simulink model "smc_AMB_digital_v2"  (R2025b)
settings: Solver=FixedStepAuto  StartTime=0.0  StopTime=2.9  FixedStep=0.0001  RelTol=1e-3
values from neighbouring files (symbols this model uses):
  a = -0.315/2    (= -0.1575)    [configura_planta_simulacao2.m]
  alpha = 0.8819    [configura_planta_simulacao2.m]
  Ar = 2*0.0077*0.0165*cos(pi/8)    [configura_planta_simulacao2.m]
  b = 0.315/2    (= 0.1575)    [configura_planta_simulacao2.m]
  Ix = 1/12*m*(L^2 +3*(dia/2)^2)    (= 0.0133460782333)    [configura_planta_simulacao2.m]
  Iy = Ix    (= 0.0133460782333)    [configura_planta_simulacao2.m]
  Iz = m*(dia/2)^2/2    (= 2.54898e-05)    [configura_planta_simulacao2.m]
  Kd_pid = 49    [configura_planta_simulacao2.m]
  Ki_pid = 4e4    (= 40000)    [configura_planta_simulacao2.m]
  Kp_pid = 1.2e4    (= 12000)    [configura_planta_simulacao2.m]
  m = 1    [configura_planta_simulacao2.m]
  mi0 = pi*4e-7    (= 1.25663706144e-06)    [configura_planta_simulacao2.m]
  n = 260    [configura_planta_simulacao2.m]    (also in plot_simu.m = round(numel(xs) * alvo/ppv))
  omega = 0    [configura_planta_simulacao2.m]
  Ts = 1e-4    (= 0.0001)    [configura_planta_simulacao2.m]    (also in smc_mancal_simulacao.m = single(1e-4))
  U = [IneS(2,3)+b*CM(2)*mT, IneS(3,1)-b*CM(1)*mT ... (first row only)    [configura_planta_simulacao2.m]
  y0 = -5e-4    (= -0.0005)    [configura_planta_simulacao2.m]
undefined symbols (not defined in the file or in its folder): magnitude
libraries: simulink x4
settings Model: NumberOfSteps=5  Creator=thaty  LastModifiedBy=thaty
settings RTWCC: GPUComputeCapability=3.5

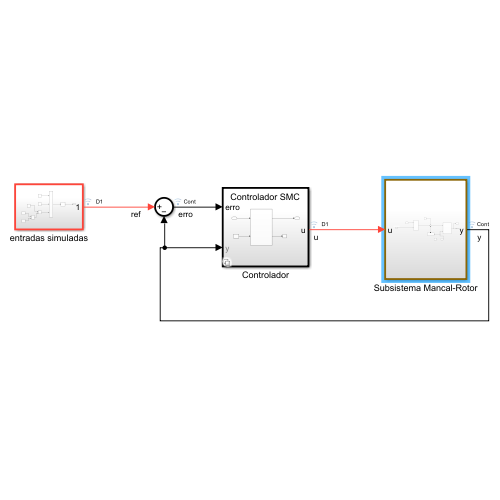
[thumbnail: Simulink's stored preview of the top-level diagram]
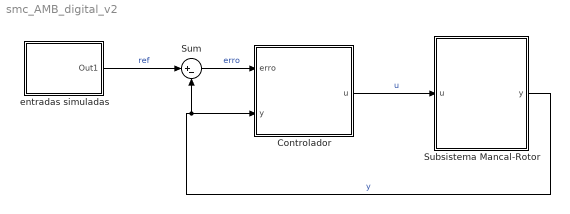
== system smc_AMB_digital_v2 ==
  Controlador : Subsystem  Variant=on
  Subsistema Mancal-Rotor : Subsystem
  Sum : Sum  Inputs=|+-
  entradas simuladas : Subsystem
  wires:
  Sum/1 -> Controlador/1(erro)  "erro"
  entradas simuladas/1(Out1) -> Sum/1  "ref"
  Subsistema Mancal-Rotor/1(y) -> Controlador/2(y), Sum/2  "y"
  Controlador/1(u) -> Subsistema Mancal-Rotor/1(u)  "u"

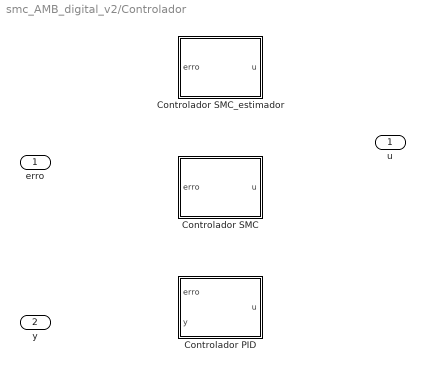
== system smc_AMB_digital_v2/Controlador ==
  erro : Inport
  y : Inport  Port=2
  Controlador PID : Subsystem  VariantControl=Type==1
  Controlador SMC : Subsystem  VariantControl=Type==2
  Controlador SMC_estimador : Subsystem  VariantControl=Type==3
  u : Outport

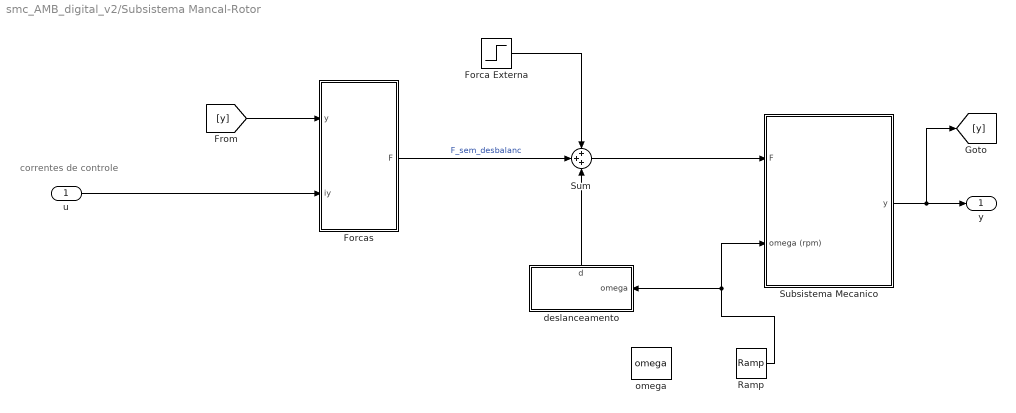
== system smc_AMB_digital_v2/Subsistema Mancal-Rotor ==
  note: correntes de controle
  u : Inport
  Forca Externa : Step  Time=2  After=0  SampleTime=0
  Forcas : Subsystem
  Ramp : simulink/Sources/Ramp  slope=10000  start=0  InitialOutput=0
  Subsistema Mecanico : Subsystem
  Sum : Sum  Inputs=+++
  deslanceamento : Subsystem
      settings: PortSchema="{\"entries\":[{\"content\":{\"sides\":[{\"content\":{},\"type\":\"ConnectorPlacement.EquallySpacedRectSide\",\"uuid\":\"45b55e67-a5ed-4805-aab1-a3da632aa8db\"},{\"content\":{\"connectorIds\":[\"In1\"],\"side\":\"RIGHT\"},\"type\":\"ConnectorPlacement.EquallySpacedRectSide\",\"uuid\":\"03c95f23-bcb1-4d33-8836-c97663662569\"},{\"content\":{\"connectorIds\":[\"Out1\"],\"side\":\"TOP\"},\"type\":\"ConnectorPlacement.EquallySpacedRectSide\",\"uuid\":\"b340f43e-95d2-40b9-ae6d-e83cbb66ff43\"}]},\"type\":\"ConnectorPlacement.EquallySpacedConnector\",\"uuid\":\"389c9e54-a030-42d8-804b-2d0e7948bbc4\"}],\"packageUris\":[\"http://schema.mathworks.com/mf0/Connector/R2020b\"],\"version\":\"1.0\"}"
  omega : Constant  Value=omega
  y : Outport
  wires:
  [y] -> Forcas/1(y)
  Forcas/1(F) -> Sum/2  "F_sem_desbalanc"
  Sum/1 -> Subsistema Mecanico/1(F)
  deslanceamento/1(d) -> Sum/3
  Subsistema Mecanico/1(y) -> [y], y/1
  Forca Externa/1 -> Sum/1
  Ramp/1 -> deslanceamento/1(omega), Subsistema Mecanico/2(omega (rpm))
  u/1 -> Forcas/2(iy)

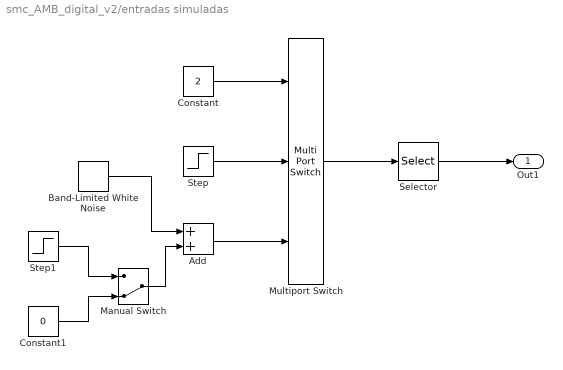
== system smc_AMB_digital_v2/entradas simuladas ==
  Add : Sum
  Band-Limited White Noise : simulink/Sources/Band-Limited White Noise  Cov=1e-14  Ts=0.0001  seed=[23341]
  Constant : Constant  Value=2
  Constant1 : Constant  Value=0
  Manual Switch : ManualSwitch  CurrentSetting=0
  Multiport Switch : MultiPortSwitch  Inputs=2  SaturateOnIntegerOverflow=off  InputSameDT=off
  Selector : Selector  InputPortWidth=1  IndexOptions=Index vector (dialog)  Indices=[1 1 1 1]  OutputSizes=1
  Step : Step  Before=y0  After=0  SampleTime=0.0001
  Step1 : Step  Before=y0  After=0  SampleTime=0.0001
  Out1 : Outport
  wires:
  Multiport Switch/1 -> Selector/1
  Band-Limited White Noise/1 -> Add/1
  Step/1 -> Multiport Switch/2
  Constant/1 -> Multiport Switch/1
  Add/1 -> Multiport Switch/3
  Selector/1 -> Out1/1
  Step1/1 -> Manual Switch/1
  Manual Switch/1 -> Add/2
  Constant1/1 -> Manual Switch/2

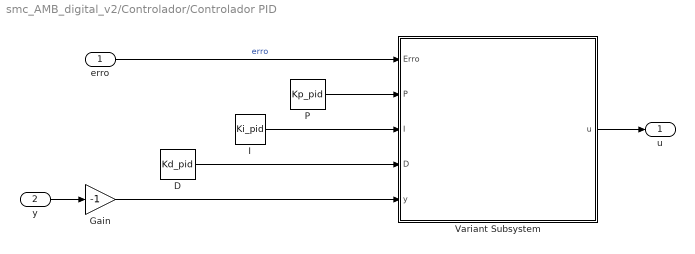
== system smc_AMB_digital_v2/Controlador/Controlador PID ==
  erro : Inport
  y : Inport  Port=2
  D : Constant  Value=Kd_pid
  Gain : Gain  Gain=-1
  I : Constant  Value=Ki_pid
  P : Constant  Value=Kp_pid
  Variant Subsystem : Subsystem  Variant=on
  u : Outport
  wires:
  y/1 -> Gain/1
  erro/1 -> Variant Subsystem/1(Erro)  "erro"
  Gain/1 -> Variant Subsystem/5(y)
  P/1 -> Variant Subsystem/2(P)
  I/1 -> Variant Subsystem/3(I)
  D/1 -> Variant Subsystem/4(D)
  Variant Subsystem/1(u) -> u/1

== system smc_AMB_digital_v2/Controlador/Controlador SMC ==
  erro : Inport
  MATLAB Function : MATLAB Function  TreatAsAtomicUnit=on
  Terminator : Terminator
  c : Constant
  u : Outport
  wires:
  c/1 -> MATLAB Function/2(enable)
  MATLAB Function/1(i_ctrl) -> u/1  "corrente_controle"
  erro/1 -> MATLAB Function/1(erro)  "posicao"
  MATLAB Function/2(s_out) -> Terminator/1  "superficie"

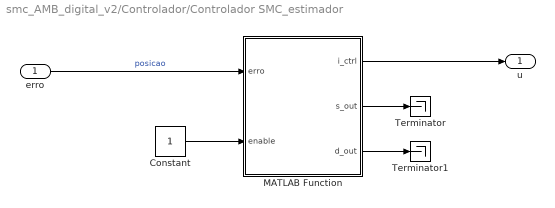
== system smc_AMB_digital_v2/Controlador/Controlador SMC_estimador ==
  erro : Inport
  Constant : Constant
  MATLAB Function : MATLAB Function  TreatAsAtomicUnit=on
  Terminator : Terminator
  Terminator1 : Terminator
  u : Outport
  wires:
  erro/1 -> MATLAB Function/1(erro)  "posicao"
  MATLAB Function/1(i_ctrl) -> u/1
  Constant/1 -> MATLAB Function/2(enable)
  MATLAB Function/3(d_out) -> Terminator1/1
  MATLAB Function/2(s_out) -> Terminator/1

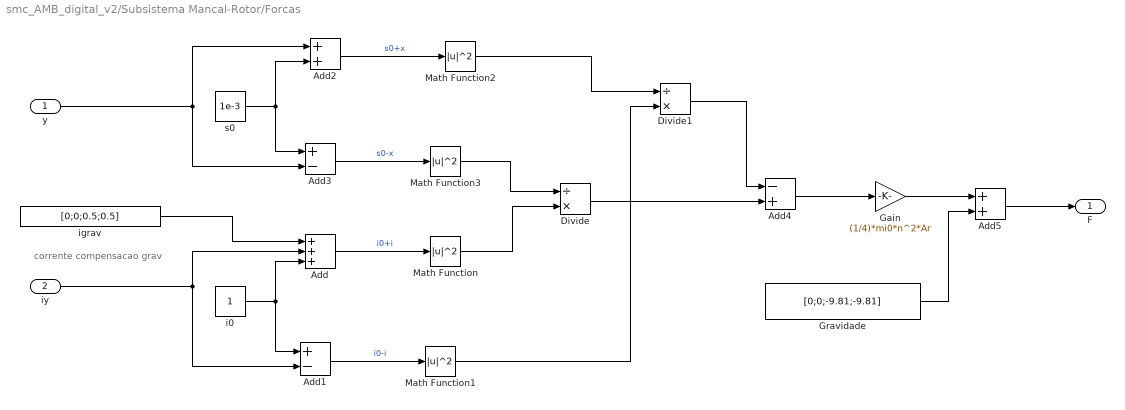
== system smc_AMB_digital_v2/Subsistema Mancal-Rotor/Forcas ==
  note: corrente compensacao grav
  y : Inport
  iy : Inport  Port=2
  Add : Sum  Inputs=+++
  Add1 : Sum  Inputs=+-
  Add2 : Sum
  Add3 : Sum  Inputs=+-
  Add4 : Sum  Inputs=-+
  Add5 : Sum
  Divide : Product  Inputs=/*
  Divide1 : Product  Inputs=/*
  Gain : Gain  Gain=(1/4)*mi0*n^2*Ar
  Gravidade : Constant  Value=[0;0;-9.81;-9.81]
  Math Function{,1..3} (4 alike) : Math  Operator=magnitude^2  SignedPower=on  RndMeth=Zero
  i0 : Constant
  igrav : Constant  Value=[0;0;0.5;0.5]
  s0 : Constant  Value=1e-3
  F : Outport
  wires:
  y/1 -> Add2/1, Add3/2
  Add3/1 -> Math Function3/1  "s0-x"
  s0/1 -> Add3/1, Add2/2
  Add2/1 -> Math Function2/1  "s0+x"
  Add/1 -> Math Function/1  "i0+i"
  i0/1 -> Add/3, Add1/1
  Add1/1 -> Math Function1/1  "i0-i"
  Math Function3/1 -> Divide/1
  Math Function/1 -> Divide/2
  Math Function2/1 -> Divide1/1
  Math Function1/1 -> Divide1/2
  Add4/1 -> Gain/1
  Divide1/1 -> Add4/1
  Gain/1 -> Add5/1
  Add5/1 -> F/1
  Divide/1 -> Add4/2
  iy/1 -> Add1/2, Add/2
  igrav/1 -> Add/1
  Gravidade/1 -> Add5/2

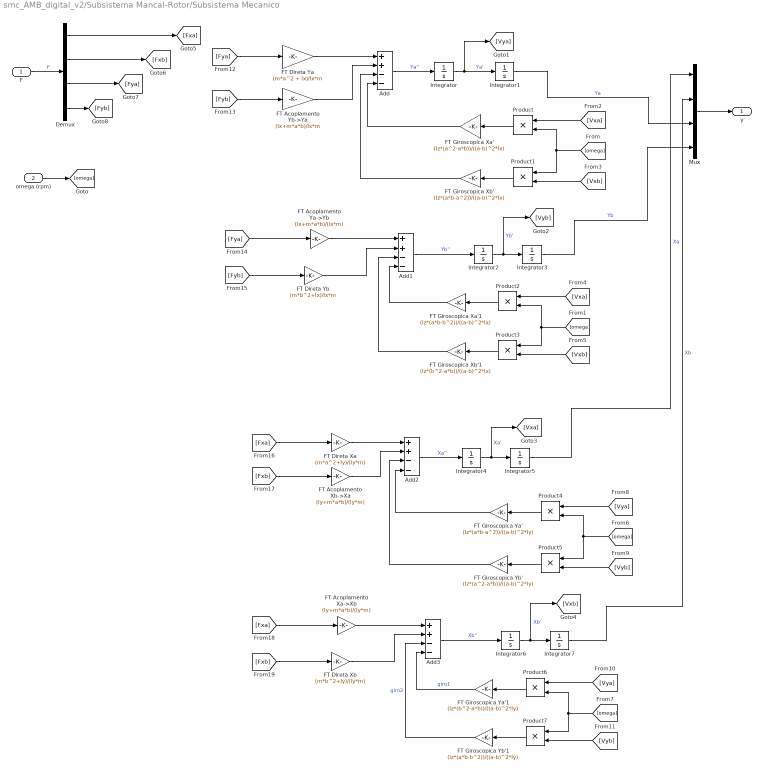
== system smc_AMB_digital_v2/Subsistema Mancal-Rotor/Subsistema Mecanico ==
  F : Inport
  omega (rpm) : Inport  Port=2
  Add{,1..3} (4 alike) : Sum  Inputs=++--
  Demux : Demux
  FT Acoplamento Xa->Xb : Gain  Gain=(Iy+m*a*b)/(Iy*m)
  FT Acoplamento Xb->Xa : Gain  Gain=(Iy+m*a*b)/(Iy*m)
  FT Acoplamento Ya->Yb : Gain  Gain=(Ix+m*a*b)/(Ix*m)
  FT Acoplamento Yb->Ya : Gain  Gain=(Ix+m*a*b)/Ix*m
  FT Direta Xa : Gain  Gain=(m*a^2+Iy)/(Iy*m)
  FT Direta Xb : Gain  Gain=(m*b^2+Iy)/(Iy*m)
  FT Direta Ya : Gain  Gain=(m*a^2 + Ix)/Ix*m
  FT Direta Yb : Gain  Gain=(m*b^2+Ix)/Ix*m
  FT Giroscopica Xa' : Gain  Gain=(Iz*(a^2-a*b))/((a-b)^2*Ix)
  FT Giroscopica Xa'1 : Gain  Gain=(Iz*(a*b-b^2))/((a-b)^2*Ix)
  FT Giroscopica Xb' : Gain  Gain=(Iz*(a*b-a^2))/((a-b)^2*Ix)
  FT Giroscopica Xb'1 : Gain  Gain=(Iz*(b^2-a*b))/((a-b)^2*Ix)
  FT Giroscopica Ya' : Gain  Gain=(Iz*(a*b-a^2))/((a-b)^2*Iy)
  FT Giroscopica Ya'1 : Gain  Gain=(Iz*(b^2-a*b))/((a-b)^2*Iy)
  FT Giroscopica Yb' : Gain  Gain=(Iz*(a^2-a*b))/((a-b)^2*Iy)
  FT Giroscopica Yb'1 : Gain  Gain=(Iz*(a*b-b^2))/((a-b)^2*Iy)
  Integrator{,1..7} (8 alike) : Integrator  InitialCondition=y0
  Mux : Mux
  Product{,1..7} (8 alike) : Product
  y : Outport
  wires:
  omega (rpm)/1 -> [omega]
  [omega] -> Product/2, Product1/1
  Product/1 -> FT Giroscopica Xa'/1
  Product1/1 -> FT Giroscopica Xb'/1
  FT Direta Ya/1 -> Add/1
  FT Acoplamento Yb->Ya/1 -> Add/2
  FT Giroscopica Xa'/1 -> Add/4
  FT Giroscopica Xb'/1 -> Add/3
  Add/1 -> Integrator/1  "Ya''"
  Integrator/1 -> [Vya], Integrator1/1  "Ya'"
  Integrator1/1 -> Mux/3  "Ya"
  Product2/1 -> FT Giroscopica Xa'1/1
  Product3/1 -> FT Giroscopica Xb'1/1
  [omega] -> Product3/1, Product2/2
  FT Acoplamento Ya->Yb/1 -> Add1/1
  FT Direta Yb/1 -> Add1/2
  FT Giroscopica Xa'1/1 -> Add1/4
  FT Giroscopica Xb'1/1 -> Add1/3
  Integrator3/1 -> Mux/4  "Yb"
  Integrator2/1 -> [Vyb], Integrator3/1  "Yb'"
  Add1/1 -> Integrator2/1  "Yb''"
  [Vxb] -> Product1/2
  [Vxa] -> Product/1
  [Vxa] -> Product2/1
  [Vxb] -> Product3/2
  [Vyb] -> Product5/2
  [Vya] -> Product4/1
  Product6/1 -> FT Giroscopica Ya'1/1
  FT Giroscopica Ya'1/1 -> Add3/4  "giro1"
  FT Giroscopica Yb'1/1 -> Add3/3  "giro2"
  Product7/1 -> FT Giroscopica Yb'1/1
  Integrator5/1 -> Mux/1  "Xa"
  [omega] -> Product7/1, Product6/2
  FT Giroscopica Yb'/1 -> Add2/3
  Product4/1 -> FT Giroscopica Ya'/1
  [Vyb] -> Product7/2
  Integrator4/1 -> [Vxa], Integrator5/1  "Xa'"
  Integrator6/1 -> [Vxb], Integrator7/1  "Xb'"
  Add3/1 -> Integrator6/1  "Xb''"
  FT Acoplamento Xb->Xa/1 -> Add2/2
  FT Direta Xa/1 -> Add2/1
  [Vya] -> Product6/1
  FT Direta Xb/1 -> Add3/2
  Product5/1 -> FT Giroscopica Yb'/1
  Integrator7/1 -> Mux/2  "Xb"
  FT Giroscopica Ya'/1 -> Add2/4
  Add2/1 -> Integrator4/1  "Xa''"
  [omega] -> Product4/2, Product5/1
  FT Acoplamento Xa->Xb/1 -> Add3/1
  F/1 -> Demux/1  "F"
  Demux/4 -> [Fyb]
  Demux/3 -> [Fya]
  Demux/2 -> [Fxb]
  Demux/1 -> [Fxa]
  [Fya] -> FT Direta Ya/1
  [Fyb] -> FT Acoplamento Yb->Ya/1
  [Fyb] -> FT Direta Yb/1
  [Fya] -> FT Acoplamento Ya->Yb/1
  [Fxb] -> FT Acoplamento Xb->Xa/1
  [Fxa] -> FT Direta Xa/1
  [Fxb] -> FT Direta Xb/1
  [Fxa] -> FT Acoplamento Xa->Xb/1
  Mux/1 -> y/1

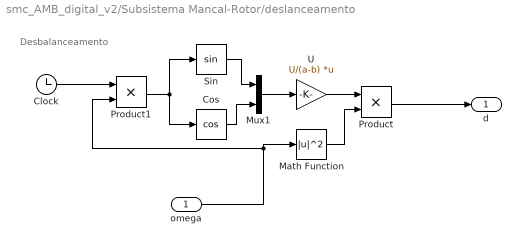
== system smc_AMB_digital_v2/Subsistema Mancal-Rotor/deslanceamento ==
  note: Desbalanceamento
  omega : Inport
  Clock : Clock
  Cos : Trigonometry  Operator=cos
  Math Function : Math  Operator=magnitude^2  SignedPower=on  RndMeth=Zero
  Mux1 : Mux  Inputs=2
  Product : Product
  Product1 : Product
  Sin : Trigonometry
  U : Gain  Gain=U/(a-b)  Multiplication=Matrix(K*u)
  d : Outport
  wires:
  Cos/1 -> Mux1/2
  Math Function/1 -> Product/2
  Product1/1 -> Cos/1, Sin/1
  Clock/1 -> Product1/1
  omega/1 -> Product1/2, Math Function/1
  U/1 -> Product/1
  Mux1/1 -> U/1
  Sin/1 -> Mux1/1
  Product/1 -> d/1

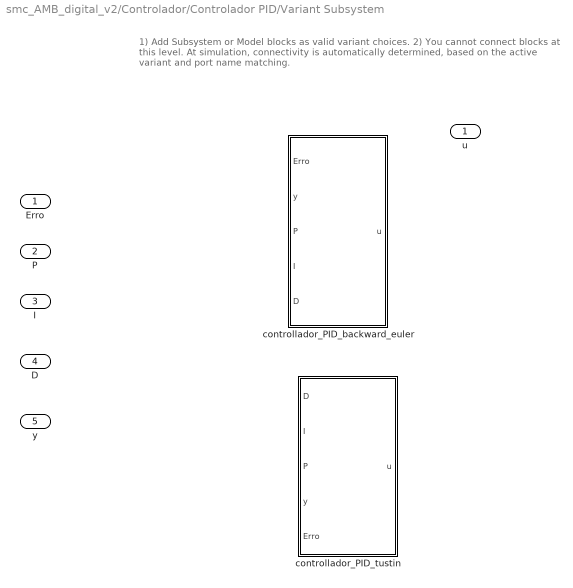
== system smc_AMB_digital_v2/Controlador/Controlador PID/Variant Subsystem ==
  note: 1) Add Subsystem or Model blocks as valid variant choices.
      | 2) You cannot connect blocks at this level. At simulation, connectivity is automatically
      | determined, based on the active variant and port name matching.
  Erro : Inport
  P : Inport  Port=2
  I : Inport  Port=3
  D : Inport  Port=4
  y : Inport  Port=5
  " controllador_PID_backward_euler" : Subsystem  VariantControl=PID_Type==1
  " controllador_PID_tustin" : Subsystem  VariantControl=PID_Type==2
  u : Outport

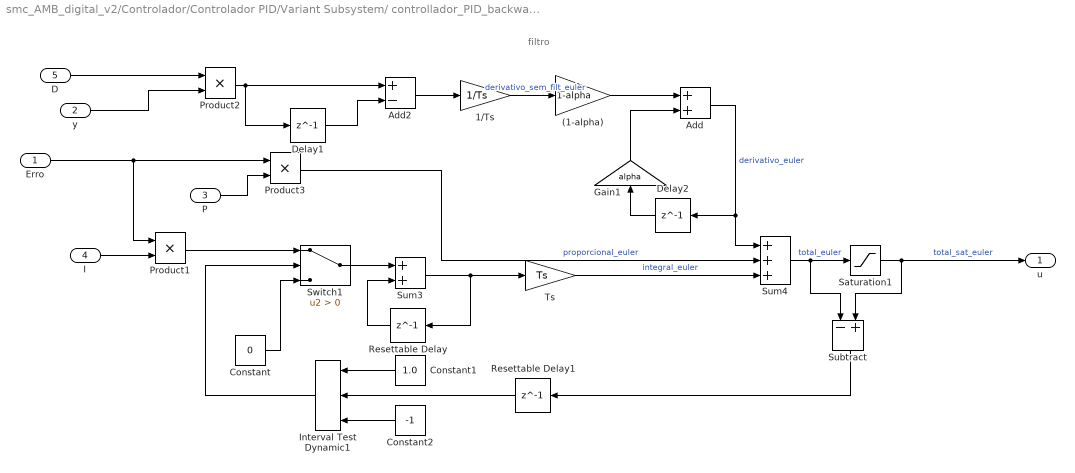
== system smc_AMB_digital_v2/Controlador/Controlador PID/Variant Subsystem/ controllador_PID_backward_euler ==
  note: filtro
  Erro : Inport
  y : Inport  Port=2
  P : Inport  Port=3
  I : Inport  Port=4
  D : Inport  Port=5
  (1-alpha) : Gain  Gain=1-alpha
  1/Ts : Gain  Gain=1/Ts  ParamDataTypeStr=single  OutDataTypeStr=single
  Add : Sum
  Add2 : Sum  Inputs=+-  OutDataTypeStr=single  AccumDataTypeStr=single
  Constant : Constant  Value=0  OutDataTypeStr=single
  Constant1 : Constant  Value=1.0  OutDataTypeStr=single
  Constant2 : Constant  Value=-1  OutDataTypeStr=single
  Delay1 : Delay  DelayLength=1
  Delay2 : Delay  DelayLength=1
  Gain1 : Gain  Gain=alpha
  Interval Test Dynamic1 : simulink/Logic and Bit Operations/Interval Test Dynamic  IntervalClosedRight=on  IntervalClosedLeft=on  OutDataTypeStr=boolean
  Product1 : Product  OutDataTypeStr=single
  Product2 : Product  OutDataTypeStr=single
  Product3 : Product  OutDataTypeStr=single
  Resettable Delay : Delay  DelayLength=1
  Resettable Delay1 : Delay  DelayLength=1
  Saturation1 : Saturate  UpperLimit=1  LowerLimit=-1
  Subtract : Sum  Inputs=-+  OutDataTypeStr=single  AccumDataTypeStr=single
  Sum3 : Sum  OutDataTypeStr=single  AccumDataTypeStr=single
  Sum4 : Sum  Inputs=+++  OutDataTypeStr=single  AccumDataTypeStr=single
  Switch1 : Switch  Criteria=u2 > Threshold  OutDataTypeStr=single  SaturateOnIntegerOverflow=off  InputSameDT=off
  Ts : Gain  Gain=Ts  ParamDataTypeStr=single  OutDataTypeStr=single
  u : Outport  VectorParamsAs1DForOutWhenUnconnected=off
  wires:
  Resettable Delay1/1 -> Interval Test Dynamic1/2
  Product3/1 -> Sum4/2  "proporcional_euler"
  Constant1/1 -> Interval Test Dynamic1/1
  Subtract/1 -> Resettable Delay1/1
  Constant/1 -> Switch1/3
  Interval Test Dynamic1/1 -> Switch1/2
  Delay1/1 -> Add2/2
  Switch1/1 -> Sum3/1
  Product2/1 -> Delay1/1, Add2/1
  I/1 -> Product1/2
  Erro/1 -> Product1/1, Product3/1
  Resettable Delay/1 -> Sum3/2
  Constant2/1 -> Interval Test Dynamic1/3
  Sum4/1 -> Saturation1/1, Subtract/1  "total_euler"
  Sum3/1 -> Resettable Delay/1, Ts/1
  Ts/1 -> Sum4/3  "integral_euler"
  Product1/1 -> Switch1/1
  Add2/1 -> 1/Ts/1
  Saturation1/1 -> Subtract/2, u/1  "total_sat_euler"
  P/1 -> Product3/2
  D/1 -> Product2/1
  1/Ts/1 -> (1-alpha)/1  "derivativo_sem_filt_euler"
  (1-alpha)/1 -> Add/1
  Add/1 -> Sum4/1, Delay2/1  "derivativo_euler"
  Delay2/1 -> Gain1/1
  Gain1/1 -> Add/2
  y/1 -> Product2/2

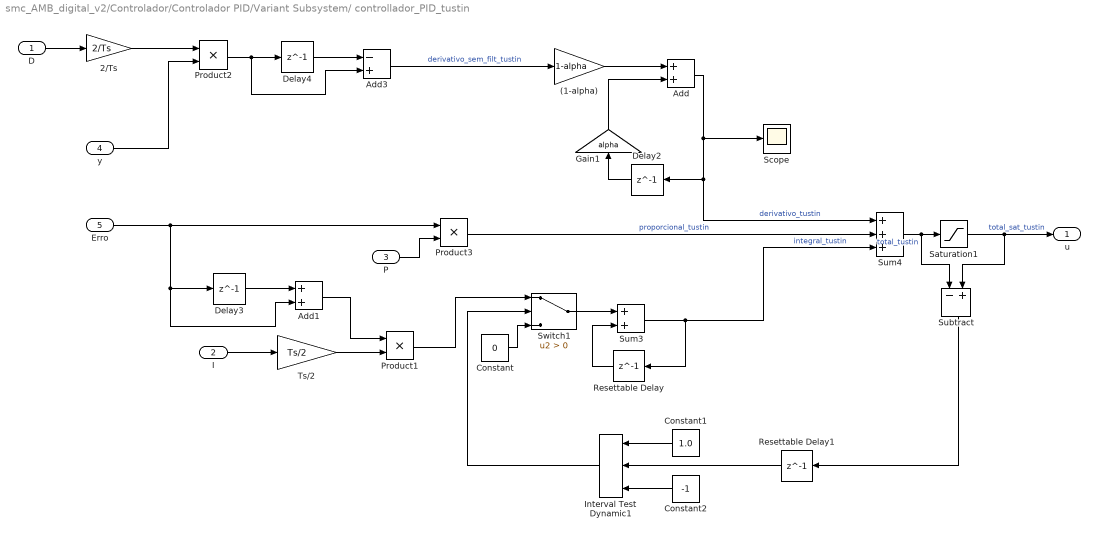
== system smc_AMB_digital_v2/Controlador/Controlador PID/Variant Subsystem/ controllador_PID_tustin ==
  D : Inport
  I : Inport  Port=2
  P : Inport  Port=3
  y : Inport  Port=4
  Erro : Inport  Port=5
  (1-alpha) : Gain  Gain=1-alpha
  2/Ts : Gain  Gain=2/Ts  ParamDataTypeStr=single  OutDataTypeStr=single
  Add : Sum
  Add1 : Sum
  Add3 : Sum  Inputs=-+
  Constant : Constant  Value=0  OutDataTypeStr=single
  Constant1 : Constant  Value=1.0  OutDataTypeStr=single
  Constant2 : Constant  Value=-1  OutDataTypeStr=single
  Delay2 : Delay  DelayLength=1  InitialCondition=y0
  Delay3 : Delay  DelayLength=1  InitialCondition=y0
  Delay4 : Delay  DelayLength=1  InitialCondition=y0
  Gain1 : Gain  Gain=alpha
  Interval Test Dynamic1 : simulink/Logic and Bit Operations/Interval Test Dynamic  IntervalClosedRight=on  IntervalClosedLeft=on  OutDataTypeStr=boolean
  Product1 : Product  OutDataTypeStr=single
  Product2 : Product  OutDataTypeStr=single
  Product3 : Product  OutDataTypeStr=single
  Resettable Delay : Delay  DelayLength=1  InitialCondition=y0
  Resettable Delay1 : Delay  DelayLength=1  InitialCondition=y0
  Saturation1 : Saturate  UpperLimit=1  LowerLimit=-1
  Scope : Scope
      settings: ActiveDisplayYMinimum=-0.69579825177788723  ActiveDisplayYMaximum=3.6245258487761021
  Subtract : Sum  Inputs=-+  OutDataTypeStr=single  AccumDataTypeStr=single
  Sum3 : Sum  OutDataTypeStr=single  AccumDataTypeStr=single
  Sum4 : Sum  Inputs=+++  OutDataTypeStr=single  AccumDataTypeStr=single
  Switch1 : Switch  Criteria=u2 > Threshold  OutDataTypeStr=single  SaturateOnIntegerOverflow=off  InputSameDT=off
  Ts/2 : Gain  Gain=Ts/2  ParamDataTypeStr=single  OutDataTypeStr=single
  u : Outport  VectorParamsAs1DForOutWhenUnconnected=off
  wires:
  Resettable Delay1/1 -> Interval Test Dynamic1/2
  Product3/1 -> Sum4/2  "proporcional_tustin"
  Constant1/1 -> Interval Test Dynamic1/1
  Subtract/1 -> Resettable Delay1/1
  Constant/1 -> Switch1/3
  Interval Test Dynamic1/1 -> Switch1/2
  Switch1/1 -> Sum3/1
  I/1 -> Ts/2/1
  Erro/1 -> Product3/1, Add1/2, Delay3/1
  Resettable Delay/1 -> Sum3/2
  Constant2/1 -> Interval Test Dynamic1/3
  Sum4/1 -> Saturation1/1, Subtract/1  "total_tustin"
  Sum3/1 -> Sum4/3, Resettable Delay/1  "integral_tustin"
  Product1/1 -> Switch1/1
  Saturation1/1 -> u/1, Subtract/2  "total_sat_tustin"
  P/1 -> Product3/2
  D/1 -> 2/Ts/1
  Add3/1 -> (1-alpha)/1  "derivativo_sem_filt_tustin"
  (1-alpha)/1 -> Add/1
  Add/1 -> Sum4/1, Delay2/1, Scope/1  "derivativo_tustin"
  Delay2/1 -> Gain1/1
  Gain1/1 -> Add/2
  Ts/2/1 -> Product1/2
  Delay3/1 -> Add1/1
  Add1/1 -> Product1/1
  2/Ts/1 -> Product2/1
  Delay4/1 -> Add3/1
  Product2/1 -> Add3/2, Delay4/1
  y/1 -> Product2/2

== matlab function smc_AMB_digital_v2/Controlador/Controlador SMC_estimador/MATLAB Function ==
  data: erro input; i_ctrl output; enable input; s_out output; d_out output
function [i_ctrl, s_out, d_out] = smc_mancal_eso(erro, enable)
%#codegen
% -----------------------------------------------------------------
% Controle por Modos Deslizantes (SMC) com ESTIMADOR DE ESTADO ESTENDIDO
% (ESO) para o mancal magnetico ativo.
%
% DIFERENCA PARA A VERSAO ANTERIOR (smc_mancal):
%   - a velocidade NAO vem mais de uma derivada filtrada do erro, e sim
%     de um observador. O sinal fica muito mais limpo.
%   - o termo RAZAO*e (cancelamento da rigidez negativa com |ks|/ki
%     escrito na mao) SUMIU. O observador ESTIMA essa forca sozinho,
%     no estado z3. Isso e o que da robustez a erro de modelo.
%
% ENTRADAS
%   erro   : 4x1 [ref - pos] em METROS, ordem [Ya; Xa; Yb; Xb]
%   enable : 0 desliga e zera os estados, 1 controla
%
% SAIDAS
%   i_ctrl : 4x1 corrente de controle comandada [A]
%   s_out  : 4x1 superficie de deslizamento          -> LOGAR
%   d_out  : 4x1 perturbacao estimada z3 [m/s^2]     -> LOGAR
%
% MODELO USADO PELO OBSERVADOR
%   e_ponto_ponto = -B*u + d
%   onde d agrupa TUDO que nao esta modelado: a rigidez negativa,
%   a gravidade, o desbalanceamento e qualquer erro de modelo.
%
%   z1 -> estimativa de e
%   z2 -> estimativa de e_ponto  (a velocidade que antes vinha da derivada)
%   z3 -> estimativa de d        (a perturbacao)
%
% LEI DE CONTROLE
%   s = z2 + C*z1 + C_I*integral(e)
%   u = ( z3 + C*z2 + C_I*z1 + K*s + EPS*sat(s/PHI) ) / B
% -----------------------------------------------------------------
 
% ===================== PARAMETROS =====================
    Ts     = single(1e-4);      % periodo de amostragem [s]
 
% --- observador (ESO)
    WO     = single(500);       % banda do observador [rad/s]
                                % 500 = bom compromisso.
                                % subir = estima mais rapido, mas amplifica ruido
                                % acima de ~2500 o observador discreto instabiliza
 
% --- superficie de deslizamento
    C      = single(300);       % inclinacao da superficie      [1/s]
    C_I    = single(5000);      % termo integral da superficie  [1/s^2]
 
% --- lei de controle
    K      = single(486);       % reaching gain                 [1/s]
    EPS    = single(35);        % ganho do termo descontinuo    [m/s^2]
    PHI    = single(0.02);      % camada limite                 [m/s]
                                % com o ESO o |s| ficou ~10x menor,
                                % entao da para apertar de 0.1 para 0.02
 
% --- modelo da planta
    B      = single(21.14);     % ki/m                          [N/(A*kg)]
 
% --- limites
    I_MAX  = single(2.0);       % saturacao da corrente         [A]
    EI_MAX = single(1.0e-5);    % limite do integrador          [m*s]
% ======================================================
 
% ganhos do observador (todos os polos em -WO)
    BO1 = 3*WO;
    BO2 = 3*WO*WO;
    BO3 = WO*WO*WO;
 
persistent z1 z2 z3 ei up
if isempty(z1)
    z1 = single(zeros(4,1));
    z2 = single(zeros(4,1));
    z3 = single(zeros(4,1));
    ei = single(zeros(4,1));
    up = single(zeros(4,1));
end
 
i_ctrl = single(zeros(4,1));
s_out  = single(zeros(4,1));
d_out  = single(zeros(4,1));
 
% ---- desabilitado: zera estados e saida
if enable < 0.5
    for j = 1:4
        z1(j) = single(erro(j));
        z2(j) = single(0);
        z3(j) = single(0);
        ei(j) = single(0);
        up(j) = single(0);
    end
    return;
end
 
% ---- um eixo de cada vez
for j = 1:4
    e = single(erro(j));
 
    % ---------- OBSERVADOR (ESO) ----------
    % inovacao: quanto o observador errou na posicao
    inov = e - z1(j);
 
    % integracao de Euler dos tres estados.
    % usa up(j) = corrente que a planta REALMENTE recebeu no passo anterior
    z1n = z1(j) + Ts*( z2(j)          + BO1*inov );
    z2n = z2(j) + Ts*( -B*up(j) + z3(j) + BO2*inov );
    z3n = z3(j) + Ts*(                    BO3*inov );
 
    z1(j) = z1n;
    z2(j) = z2n;
    z3(j) = z3n;
 
    % ---------- INTEGRAL DA SUPERFICIE ----------
    ei_try = ei(j) + Ts*e;
    if ei_try >  EI_MAX
        ei_try =  EI_MAX;
    end
    if ei_try < -EI_MAX
        ei_try = -EI_MAX;
    end
 
    % ---------- SUPERFICIE ----------
    % agora usa z2 (estimado) no lugar da derivada filtrada
    s = z2(j) + C*z1(j) + C_I*ei_try;
 
    % ---------- TERMO DESCONTINUO SUAVIZADO ----------
    r = s/PHI;
    if r >  1
        r =  single(1);
    end
    if r < -1
        r = -single(1);
    end
 
    % ---------- LEI DE CONTROLE ----------
    % z3 cancela a perturbacao estimada (faz o papel do antigo RAZAO*e)
    u = ( z3(j) + C*z2(j) + C_I*z1(j) + K*s + EPS*r ) / B;
 
    % ---------- SATURACAO + ANTI-WINDUP ----------
    if u > I_MAX
        u = I_MAX;
    elseif u < -I_MAX
        u = -I_MAX;
    else
        ei(j) = ei_try;
    end
 
    % guarda a corrente aplicada: o observador precisa dela no proximo passo
    up(j) = u;
 
    i_ctrl(j) = u;
    s_out(j)  = s;
    d_out(j)  = z3(j);
end
end

== matlab function smc_AMB_digital_v2/Controlador/Controlador SMC/MATLAB Function ==
  settings: updateMethod=DISCRETE
  data: erro input; i_ctrl output; enable input; s_out output
function [i_ctrl, s_out] = smc_mancal(erro, enable)
%#codegen
% -----------------------------------------------------------------
% Controle por Modos Deslizantes (SMC) para o mancal magnetico ativo.
%
% ENTRADAS
%   pos    : 4x1 [Ya; Xa; Yb; Xb] em METROS
%   ref    : 4x1 referencia, mesma ordem e unidade
%   enable : 0 desliga e zera os estados, 1 controla
%
% SAIDAS
%   i_ctrl : 4x1 corrente de controle comandada [A]
%   s_out  : 4x1 superficie de deslizamento     -> LOGAR
%
% Lei implementada (equivalente a eq. 4.29 do texto):
%   s = de + C*e + C_I*integral(e)
%   i = ( K*s + C*de + C_I*e + EPS*sat(s/PHI) )/B  +  RAZAO*e
%
% O ultimo termo e o cancelamento da rigidez negativa, que no texto
% aparece como f(x)/b. Usa a razao |ks|/ki medida na bancada.
% -----------------------------------------------------------------
 
% ===================== PARAMETROS =====================
    Ts     = single(1e-4);      % periodo de amostragem [s]
 
    % --- superficie de deslizamento
    C      = single(300);    % inclinacao da superficie      [1/s]
    C_I    = single(5000);     % termo integral da superficie  [1/s^2]
 
    % --- lei de controle
    K      = single(400);    % reaching gain                 [1/s]
    EPS    = single(25);         % ganho do termo descontinuo    [m/s^2]
    PHI    = single(0.1);       % camada limite                 [m/s]
 
    % --- modelo da planta
    B      = single(21.14);      % ki/m                          [N/(A*kg)]
    RAZAO  = single(1000);         % |ks|/ki do feedforward        [A/m]
 
    % --- limites
    I_MAX  = single(1.0);       % saturacao da corrente         [A]
    EI_MAX = single(0.01);      % limite do integrador          [m*s]
 
    % --- derivada filtrada em 200 Hz (Tustin), nao alterar
    BV     = single(1182.35);
    AV     = single(0.88177);
% ======================================================
 
persistent ep vf ei
if isempty(ep)
    ep = single(zeros(4,1));
    vf = single(zeros(4,1));
    ei = single(zeros(4,1));
end
 
i_ctrl = single(zeros(4,1));
s_out  = single(zeros(4,1));
 
% ---- desabilitado: zera estados e saida
if enable < 0.5
    for j = 1:4
        ep(j) = single(erro(j));
        vf(j) = single(0);
        ei(j) = single(0);
    end
    return;
end
 
% ---- um eixo de cada vez
for j = 1:4
 
    e = single(erro(j));
 
    % derivada do erro, filtrada
    vf(j) = AV*vf(j) + BV*(e - ep(j));
    ep(j) = e;
 
    % integral candidata, com limite
    ei_try = ei(j) + Ts*e;
    if ei_try >  EI_MAX
        ei_try =  EI_MAX;
    end
    if ei_try < -EI_MAX
        ei_try = -EI_MAX;
    end
 
    % superficie de deslizamento
    s = vf(j) + C*e + C_I*ei_try;
 
    % termo descontinuo suavizado: sat(s/PHI) no lugar de sign(s)
    r = s/PHI;
    if r >  1
        r =  single(1);
    end
    if r < -1
        r = -single(1);
    end
 
    % lei de controle
    u = (K*s + C*vf(j) + C_I*e + EPS*r)/B + RAZAO*e;
 
    % saturacao com anti-windup por integracao condicional
    if u > I_MAX
        u = I_MAX;
    elseif u < -I_MAX
        u = -I_MAX;
    else
        ei(j) = ei_try;
    end
 
    i_ctrl(j) = u;
    s_out(j)  = s;
end
end
